simulink model "MotorLink"  (R2020a)
settings: Solver=ode4  StartTime=0.0  StopTime=30  FixedStep=0.001  RelTol=1e-3
values from neighbouring files (symbols this model uses):
  A = [0 1 0 ... (first row only)    [initexp6.m]
  B = [0;0;1/L]    [initexp6.m]
  C = [1 0 0]    [initexp6.m]
  d = 0.1    [initexp6.m]
  D = 0    [initexp6.m]
  g = 9.81    [initexp6.m]
  h = place(A',C',q).'    [initexp6.m]
  J = 0.001    [initexp6.m]
  ke = 0.1    [initexp6.m]
  km = 0.1    [initexp6.m]
  kT = krT*inv(T)    [initexp6.m]
  L = 0.01    [initexp6.m]
  l = 0.1375    [initexp6.m]
  m = 1    [initexp6.m]
  R = 0.1    [initexp6.m]
settings Model: Creator=baradaran  LastModifiedBy=User

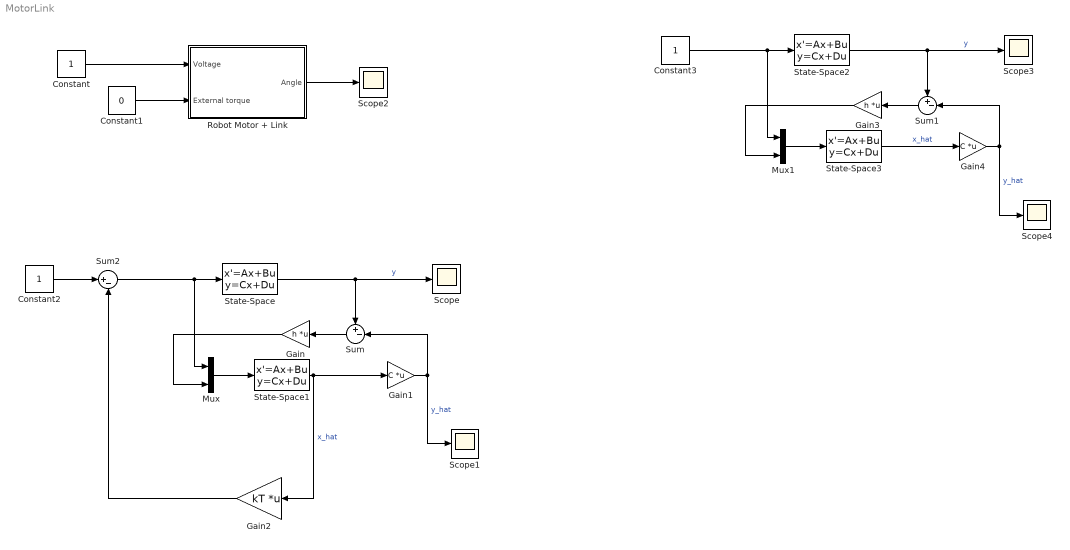
== system MotorLink ==
  Constant : Constant
  Constant1 : Constant  Value=0
  Constant2 : Constant
  Constant3 : Constant
  Gain : Gain  Gain=h  Multiplication=Matrix(K*u)
  Gain1 : Gain  Gain=C  Multiplication=Matrix(K*u)
  Gain2 : Gain  Gain=kT  Multiplication=Matrix(K*u)
  Gain3 : Gain  Gain=h  Multiplication=Matrix(K*u)
  Gain4 : Gain  Gain=C  Multiplication=Matrix(K*u)
  Mux : Mux  Inputs=2
  Mux1 : Mux  Inputs=2
  Robot Motor + Link : Subsystem  mask{J=J, ke=ke, R=R, In=L, km=km, d=d, m=m, l=l, g=g}
      mask prompts: J "Massenträgheitsmoment"; ke "elektrische Motorkonstante"; R "elektrischer Widerstand"; In "Induktivität"; km "mechanische Motorkonstante"; d "mechanische Dämpfung"; m "Gelenkmasse"; l "Massenschwerpunkt des Gelenks"; g "Gravitation"
  Scope{,1..4} (5 alike) : Scope
  State-Space : StateSpace  A=A  B=B  C=C  D=D  InitialCondition=[0;0;0]
  State-Space1 : StateSpace  A=A  B=[0 1 0 0;0 0 1 0;1/L 0 0 1];  C=[1 0 0;0 1 0;0 0 1];  D=[0 0 0 0;0 0 0 0;0 0 0 0];  InitialCondition=[0;0;0]
  State-Space2 : StateSpace  A=A  B=B  C=C  D=D  InitialCondition=[0;0;0]
  State-Space3 : StateSpace  A=A  B=[0 1 0 0;0 0 1 0;1/L 0 0 1];  C=[1 0 0;0 1 0;0 0 1];  D=[0 0 0 0;0 0 0 0;0 0 0 0];  InitialCondition=[0;0;0]
  Sum : Sum  Inputs=+-|
  Sum1 : Sum  Inputs=+-|
  Sum2 : Sum  Inputs=|+-
  wires:
  Constant/1 -> Robot Motor + Link/1(Voltage)
  Constant1/1 -> Robot Motor + Link/2(External torque)
  State-Space/1 -> Scope/1, Sum/1  "y"
  Sum/1 -> Gain/1
  Gain/1 -> Mux/2
  Mux/1 -> State-Space1/1
  State-Space1/1 -> Gain2/1, Gain1/1  "x_hat"
  Robot Motor + Link/1(Angle) -> Scope2/1
  Gain1/1 -> Scope1/1, Sum/2  "y_hat"
  Constant2/1 -> Sum2/1
  Gain2/1 -> Sum2/2
  Sum2/1 -> Mux/1, State-Space/1
  Constant3/1 -> Mux1/1, State-Space2/1
  Gain4/1 -> Scope4/1, Sum1/2  "y_hat"
  State-Space3/1 -> Gain4/1  "x_hat"
  Mux1/1 -> State-Space3/1
  Gain3/1 -> Mux1/2
  Sum1/1 -> Gain3/1
  State-Space2/1 -> Scope3/1, Sum1/1  "y"

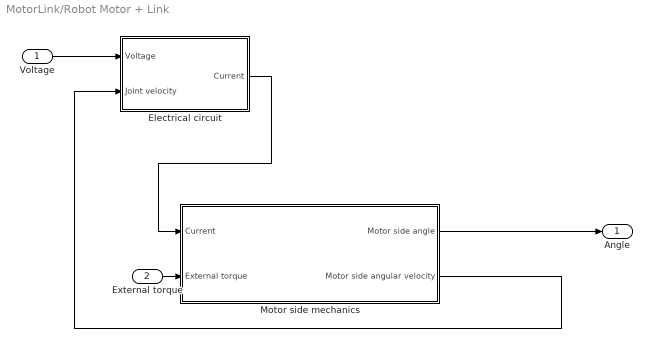
== system MotorLink/Robot Motor + Link ==
  Voltage : Inport
  External torque : Inport  Port=2
  Electrical circuit : Subsystem
  Motor side mechanics : Subsystem
  Angle : Outport  VectorParamsAs1DForOutWhenUnconnected=off
  wires:
  External torque/1 -> Motor side mechanics/2(External torque)
  Motor side mechanics/1(Motor side angle) -> Angle/1
  Motor side mechanics/2(Motor side angular velocity) -> Electrical circuit/2(Joint velocity)
  Electrical circuit/1(Current) -> Motor side mechanics/1(Current)
  Voltage/1 -> Electrical circuit/1(Voltage)

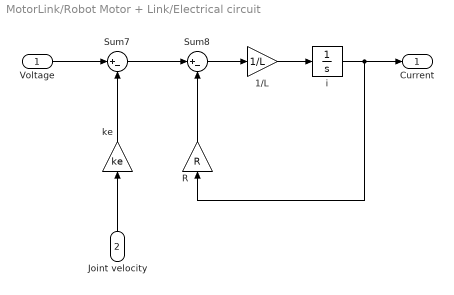
== system MotorLink/Robot Motor + Link/Electrical circuit ==
  Voltage : Inport
  Joint velocity : Inport  Port=2
  1/L : Gain  Gain=1/L
  R : Gain  Gain=R
  Sum7 : Sum  Inputs=|+-
  Sum8 : Sum  Inputs=|+-
  i : Integrator
  ke : Gain  Gain=ke
  Current : Outport  VectorParamsAs1DForOutWhenUnconnected=off
  wires:
  Sum7/1 -> Sum8/1
  i/1 -> R/1, Current/1
  R/1 -> Sum8/2
  Voltage/1 -> Sum7/1
  Joint velocity/1 -> ke/1
  ke/1 -> Sum7/2
  Sum8/1 -> 1/L/1
  1/L/1 -> i/1

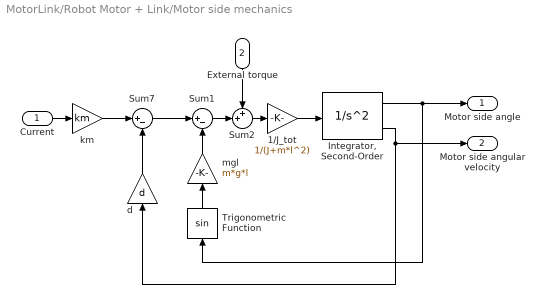
== system MotorLink/Robot Motor + Link/Motor side mechanics ==
  Current : Inport
  External torque : Inport  Port=2
  1/J_tot : Gain  Gain=1/(J+m*l^2)
  "Integrator, Second-Order" : SecondOrderIntegrator
  Sum1 : Sum  Inputs=|+-
  Sum2 : Sum  Inputs=++|
  Sum7 : Sum  Inputs=|+-
  Trigonometric Function : Trigonometry
  d : Gain  Gain=d
  km : Gain  Gain=km
  mgl : Gain  Gain=m*g*l
  Motor side angle : Outport  VectorParamsAs1DForOutWhenUnconnected=off
  Motor side angular velocity : Outport  Port=2  VectorParamsAs1DForOutWhenUnconnected=off
  wires:
  External torque/1 -> Sum2/1
  Sum1/1 -> Sum2/2
  Sum2/1 -> 1/J_tot/1
  Trigonometric Function/1 -> mgl/1
  Current/1 -> km/1
  "Integrator, Second-Order"/2 -> d/1, Motor side angular velocity/1
  1/J_tot/1 -> "Integrator, Second-Order"/1
  "Integrator, Second-Order"/1 -> Motor side angle/1, Trigonometric Function/1
  Sum7/1 -> Sum1/1
  mgl/1 -> Sum1/2
  d/1 -> Sum7/2
  km/1 -> Sum7/1
